simulink model "Electrical_System_2018b_obfs"  (R2019b)
settings: Solver=VariableStepAuto  StartTime=0.0  StopTime=5  RelTol=1e-3  AbsTol=1e-3  EnableMultiTasking=on
InitFcn:
  | Steady_State_Initialisation;
StopFcn:
  | %sscexplore(simlog);
  | %Logging
undefined symbols (not defined in the file): abrlhklxvp, aexgmhuedq, afmfmjnutg, afpphrjpnc, ahuxbyvruc, alarvljztt, amxnyqmnuw, aodrlwvqie, aolhmuplyq, aqpmguuqkg, auesgwirzl, aurophlnng, awamelrhru, ayfhvxflxn, azxkacuhqc, babszerikg, bawhdqanwq, bevoqecvei, bltjvqbchx, bmqsuewujl, bsmyqjfgnf, btvjbsmnve, bywgxqeadw, bziaduxaer, bzmcmdqocb, bzsvyvetat, ccsjnrbsih, cdvenygxwh, cedkrnslhx, cjheorclzs, cjrdshrtqx, ckhavyhcza, ckxewznhlz, cmrcgyiplk, conenicnws, cqkejbgjnn, csfnuwymhe, cunupkhwbh, cwzfvzuxxh, dcadmadufn, dcfponivnv, ddtrqjrhjn, dfhoxvkqas, dfrhtcwpne, dfvomcagjv, djijwylxea, dnmeqksrrm, dnzewbdkaa, dsqcykyxav, dtswwlttmm, ecumpidjtv, edegaywrct, ejjjsmnejc, eknqnehjdz, emvdetzouf, esxbqkbahr, etnkkbreiq, eunoiiiirw, ewewcuedir, fatkfxdhtc ... (+386)
libraries: fl_lib x802, ee_lib x362, fl_ps_legacy_lib x160, nesl_utility x85
(part 4 of 26)

== system Electrical_System_2018b_obfs/Redacted_4814/Redacted_3928/Redacted_4232 ==
  Redacted_1449 : fl_lib/Physical Signals/Sources/PS Constant  constant=eqnibszxct
  Redacted_{2466,4876,8538,9927} (4 alike) : nesl_utility/Solver Configuration  PhysicalDomain=network_engine_domain  SubClassName=solver  LeftPortType=input  RightPortType=generic  Tones=[]  Harmonics=[]  SimulateNoise=off  Profile=off  UseLocalSampling=off  EnableSwitchedLinearOptims=on  FrequencyDomain=off  UseCCode=off  RelTol=0.001  AbsTol=1e-06  MinStep=1e-09  ToWorkspace=off  RevertToSquareIcSolve=off  NumHomotopyIterations=100  PhasorMode=off  PhasorModeNumHarmonics=1  DoDC=off  ResidualTolerance=1e-09  UseLocalSolver=off  LocalSolverChoice=NE_BACKWARD_EULER_ADVANCER  LocalSolverSampleTime=0.001  DoFixedCost=off  MaxNonlinIter=3  MaxModeIter=2  LinearAlgebra=auto  EquationFormulation=NE_TIME_EF  DelaysMemoryBudget=1024  AutomaticFiltering=on  FilteringTimeConstant=0.001  PartitionStorageMethod=AS_NEEDED  PartitionMemoryBudget=1024  PartitionMethod=ROBUST
  Redacted_3160 : fl_lib/Physical Signals/Sources/PS Constant  constant=pqncstflsc
  Redacted_3437 : fl_lib/Mechanical/Mechanical Sources/Ideal Angular Velocity Source
  Redacted_4262 : fl_lib/Physical Signals/Sources/PS Constant  constant=oqqdmjcrcw
  Redacted_4413 : fl_lib/Physical Signals/Sources/PS Constant  constant=hhihvjdfsh
  Redacted_5160 : fl_lib/Mechanical/Mechanical Sources/Ideal Angular Velocity Source
  Redacted_6287 : fl_lib/Mechanical/Rotational Elements/Mechanical Rotational Reference
  Redacted_6471 : fl_lib/Gas/Elements/Controlled Reservoir (G)  area_A=txuumigmxg m^2
      settings: SourceProductName=Simscape  SourceProductBaseCode=SS  InternalSimscapePortConfiguration="{\"Bottom\":[],\"Left\":[{\"id\":\"A\",\"label\":\"A\",\"type\":\"foundation.gas.gas\"}],\"Right\":[{\"id\":\"T_in\",\"label\":\"T\",\"type\":\"input\"},{\"id\":\"p_in\",\"label\":\"P\",\"type\":\"input\"}],\"Top\":[]}"
  Redacted_6500 : fl_lib/Mechanical/Rotational Elements/Mechanical Rotational Reference
  Redacted_6772 : fl_lib/Physical Signals/Sources/PS Constant  constant=ksqpiswnhf
  Redacted_7758 : fl_lib/Gas/Elements/Controlled Reservoir (G)  area_A=bquqgacvwd m^2
      settings: SourceProductName=Simscape  SourceProductBaseCode=SS  InternalSimscapePortConfiguration="{\"Bottom\":[],\"Left\":[{\"id\":\"A\",\"label\":\"A\",\"type\":\"foundation.gas.gas\"}],\"Right\":[{\"id\":\"T_in\",\"label\":\"T\",\"type\":\"input\"},{\"id\":\"p_in\",\"label\":\"P\",\"type\":\"input\"}],\"Top\":[]}"
  Redacted_7870 : fl_lib/Physical Signals/Sources/PS Constant  constant=kaibuegcpr
  Redacted_8727 : PMIOPort  Side=Right
  Redacted_8285 : PMIOPort  Port=2  Side=Right
  Redacted_5217 : PMIOPort  Port=3  Side=Right
  Redacted_9547 : PMIOPort  Port=4  Side=Right
  connections:
  Redacted_3437/LConn1 -- Redacted_4876/RConn1 -- Redacted_5217/RConn1
  Redacted_8727/RConn1 -- Redacted_2466/RConn1 -- Redacted_5160/LConn1
  Redacted_6471/LConn1 -- Redacted_8538/RConn1 -- Redacted_8285/RConn1
  Redacted_9547/RConn1 -- Redacted_9927/RConn1 -- Redacted_7758/LConn1
  Redacted_6500/LConn1 -- Redacted_3437/RConn2
  Redacted_4413/RConn1 -- Redacted_3437/RConn1
  Redacted_5160/RConn1 -- Redacted_3160/RConn1
  Redacted_6287/LConn1 -- Redacted_5160/RConn2
  Redacted_6471/RConn2 -- Redacted_7870/RConn1
  Redacted_6471/RConn1 -- Redacted_4262/RConn1
  Redacted_7758/RConn2 -- Redacted_1449/RConn1
  Redacted_6772/RConn1 -- Redacted_7758/RConn1

== system Electrical_System_2018b_obfs/Redacted_9930/Redacted_3896/Redacted_7665 ==
  Redacted_644 : Outport  InitialOutput=Redacted 0.51183  OutputWhenUnconnectedValue=Redacted 0.067631
  Redacted_2723 : Outport  Port=2  InitialOutput=Redacted 0.06929  OutputWhenUnconnectedValue=Redacted 0.56439
  Redacted_8075 : Outport  Port=3  InitialOutput=Redacted 0.75636  OutputWhenUnconnectedValue=Redacted 0.74779
  Redacted_4126 : Outport  Port=4  InitialOutput=Redacted 0.41895  OutputWhenUnconnectedValue=Redacted 0.34397
  Redacted_7964 : Outport  Port=5  InitialOutput=Redacted 0.88105  OutputWhenUnconnectedValue=Redacted 0.087418
  Redacted_8682 : Outport  Port=6  InitialOutput=Redacted 0.94151  OutputWhenUnconnectedValue=Redacted 0.65364
  Redacted_6320 : Outport  Port=7  InitialOutput=Redacted 0.29985  OutputWhenUnconnectedValue=Redacted 0.09099
  Redacted_340 : Outport  Port=8  InitialOutput=Redacted 0.82117  OutputWhenUnconnectedValue=Redacted 0.22286
  Redacted_2756 : Outport  Port=9  InitialOutput=Redacted 0.3279  OutputWhenUnconnectedValue=Redacted 0.6909
  Redacted_3273 : Outport  Port=10  InitialOutput=Redacted 0.21327  OutputWhenUnconnectedValue=Redacted 0.44752
  Redacted_4657 : Outport  Port=11  InitialOutput=Redacted 0.58417  OutputWhenUnconnectedValue=Redacted 0.30551
  Redacted_3395 : Outport  Port=12  InitialOutput=Redacted 0.23044  OutputWhenUnconnectedValue=Redacted 0.049881
  Redacted_9977 : Outport  Port=13  InitialOutput=Redacted 0.37016  OutputWhenUnconnectedValue=Redacted 0.4867
  Redacted_2599 : Outport  Port=14  InitialOutput=Redacted 0.51394  OutputWhenUnconnectedValue=Redacted 0.10668
  Redacted_1407 : Outport  Port=15  InitialOutput=Redacted 0.046125  OutputWhenUnconnectedValue=Redacted 0.14256
  Redacted_9412 : Outport  Port=16  InitialOutput=Redacted 0.90574  OutputWhenUnconnectedValue=Redacted 0.5736
  Redacted_123 : Outport  Port=17  InitialOutput=Redacted 0.33232  OutputWhenUnconnectedValue=Redacted 0.9768
  Redacted_8209 : Outport  Port=18  InitialOutput=Redacted 0.81768  OutputWhenUnconnectedValue=Redacted 0.20788
  Redacted_531 : Outport  Port=19  InitialOutput=Redacted 0.15823  OutputWhenUnconnectedValue=Redacted 0.1958
  Redacted_6389 : Outport  Port=20  InitialOutput=Redacted 0.98917  OutputWhenUnconnectedValue=Redacted 0.89809
  Redacted_6836 : Outport  Port=21  InitialOutput=Redacted 0.049052  OutputWhenUnconnectedValue=Redacted 0.96153
  Redacted_5007 : Outport  Port=22  InitialOutput=Redacted 0.54549  OutputWhenUnconnectedValue=Redacted 0.87328
  Redacted_6497 : Outport  Port=23  InitialOutput=Redacted 0.97589  OutputWhenUnconnectedValue=Redacted 0.47787
  Redacted_9632 : Outport  Port=24  InitialOutput=Redacted 0.61016  OutputWhenUnconnectedValue=Redacted 0.8766
  Redacted_2902 : Outport  Port=25  InitialOutput=Redacted 0.56898  OutputWhenUnconnectedValue=Redacted 0.30275
  Redacted_2695 : Outport  Port=26  InitialOutput=Redacted 0.96136  OutputWhenUnconnectedValue=Redacted 0.057162
  Redacted_8396 : Outport  Port=27  InitialOutput=Redacted 0.63483  OutputWhenUnconnectedValue=Redacted 0.36709
  Redacted_9164 : Outport  Port=28  InitialOutput=Redacted 0.81001  OutputWhenUnconnectedValue=Redacted 0.29306
  Redacted_9075 : Outport  Port=29  InitialOutput=Redacted 0.54526  OutputWhenUnconnectedValue=Redacted 0.14115
  Redacted_6090 : Outport  Port=30  InitialOutput=Redacted 0.7708  OutputWhenUnconnectedValue=Redacted 0.55418

== system Electrical_System_2018b_obfs/Redacted_9930/Redacted_4814/Redacted_6431 ==
  Redacted_6479 : Outport
  Redacted_3532 : Outport  Port=2
  Redacted_6579 : Outport  Port=3
  Redacted_5091 : Outport  Port=4
  Redacted_5066 : Outport  Port=5
  Redacted_2648 : Outport  Port=6
  Redacted_3799 : Outport  Port=7
  Redacted_988 : Outport  Port=8
  Redacted_4741 : Outport  Port=9
  Redacted_474 : Outport  Port=10
  Redacted_4041 : Outport  Port=11
  Redacted_9998 : Outport  Port=12
  Redacted_2742 : Outport  Port=13
  Redacted_5781 : Outport  Port=14
  Redacted_125 : Outport  Port=15
  Redacted_4308 : Outport  Port=16
  Redacted_8077 : Outport  Port=17
  Redacted_7701 : Outport  Port=18
  Redacted_8967 : Outport  Port=19
  Redacted_8464 : Outport  Port=20
  Redacted_1093 : Outport  Port=21
  Redacted_1950 : Outport  Port=22
  Redacted_1167 : Outport  Port=23
  Redacted_3969 : Outport  Port=24
  Redacted_1905 : Outport  Port=25
  Redacted_1688 : Outport  Port=26
  Redacted_6009 : Outport  Port=27
  Redacted_9612 : Outport  Port=28
  Redacted_8082 : Outport  Port=29
  Redacted_1556 : Outport  Port=30

== system Electrical_System_2018b_obfs/Redacted_1221/Redacted_346/Redacted_2722/Redacted_9748 ==
  note: Transient
  note: Steady-State
  Redacted_8203 : Inport
  Redacted_2737 : Subsystem  VariantControl=Variant1
  Redacted_8358 : PMIOPort  Side=Left
  Redacted_4914 : PMIOPort  Port=2  Side=Left
  Redacted_5870 : PMIOPort  Port=3  Side=Left
  Redacted_79 : PMIOPort  Port=4  Side=Left
  Redacted_7076 : PMIOPort  Port=5  Side=Left
  Redacted_2739 : PMIOPort  Port=6  Side=Left
  Redacted_5893 : PMIOPort  Port=7  Side=Right
  Redacted_5379 : PMIOPort  Port=8  Side=Right
  Redacted_7574 : PMIOPort  Port=9  Side=Right
  Redacted_8270 : PMIOPort  Port=10  Side=Right
  Redacted_8085 : Outport

== system Electrical_System_2018b_obfs/Redacted_1221/Redacted_346/Redacted_3067/Redacted_5519 ==
  note: Steady State
  note: Transient
  Redacted_7936 : Inport
  Redacted_4492 : Subsystem  VariantControl=Choice
  Redacted_7038 : PMIOPort  Side=Right
  Redacted_4138 : PMIOPort  Port=2  Side=Right
  Redacted_4230 : PMIOPort  Port=3  Side=Right
  Redacted_2273 : PMIOPort  Port=4  Side=Left
  Redacted_2496 : PMIOPort  Port=5  Side=Left
  Redacted_4854 : Outport

== system Electrical_System_2018b_obfs/Redacted_1221/Redacted_346/Redacted_5295/Redacted_9981 ==
  note: Steady State
  note: Transient
  Redacted_3927 : Inport
  HP_Generation_Steady_State_Custom_Block : Subsystem  VariantControl=Choice_1
  Redacted_313 : Subsystem  VariantControl=Choice
  Redacted_2793 : PMIOPort  Side=Right
  Redacted_4361 : PMIOPort  Port=2  Side=Right
  Redacted_664 : PMIOPort  Port=3  Side=Right
  Redacted_7849 : PMIOPort  Port=4  Side=Left
  Redacted_6560 : PMIOPort  Port=5  Side=Left
  Redacted_2300 : PMIOPort  Port=6  Side=Left
  Redacted_8917 : PMIOPort  Port=7  Side=Left
  Redacted_8702 : Outport

== system Electrical_System_2018b_obfs/Redacted_1221/Redacted_346/Redacted_6610/Redacted_2835 ==
  note: Steady State
  note: Transient
  Redacted_1740 : Inport
  LP_Generation_Steady_State_Custom_Block : Subsystem  VariantControl=Choice_1
  Redacted_9252 : Subsystem  VariantControl=Choice
  Redacted_9392 : PMIOPort  Side=Right
  Redacted_5211 : PMIOPort  Port=2  Side=Right
  Redacted_1737 : PMIOPort  Port=3  Side=Right
  Redacted_5882 : PMIOPort  Port=4  Side=Left
  Redacted_3815 : PMIOPort  Port=5  Side=Left
  Redacted_3823 : PMIOPort  Port=6  Side=Left
  Redacted_270 : PMIOPort  Port=7  Side=Left
  Redacted_5993 : Outport

== system Electrical_System_2018b_obfs/Redacted_1221/Redacted_7523/Redacted_2432/Redacted_3397 ==
  note: Steady State
  note: Transient
  Redacted_7824 : Inport
  Redacted_440 : Subsystem  VariantControl=Choice
  Redacted_9237 : PMIOPort  Side=Right
  Redacted_7902 : PMIOPort  Port=2  Side=Right
  Redacted_6078 : PMIOPort  Port=3  Side=Right
  Redacted_5254 : PMIOPort  Port=4  Side=Left
  Redacted_3960 : PMIOPort  Port=5  Side=Left
  Redacted_3107 : Outport

== system Electrical_System_2018b_obfs/Redacted_1221/Redacted_7523/Redacted_5456/Redacted_1170 ==
  note: Steady State
  note: Transient
  Redacted_533 : Inport
  HP_Generation_Steady_State_Custom_Block : Subsystem  VariantControl=Choice_1
  Redacted_7838 : Subsystem  VariantControl=Choice
  Redacted_7127 : PMIOPort  Side=Right
  Redacted_9296 : PMIOPort  Port=2  Side=Right
  Redacted_1514 : PMIOPort  Port=3  Side=Right
  Redacted_8915 : PMIOPort  Port=4  Side=Left
  Redacted_4767 : PMIOPort  Port=5  Side=Left
  Redacted_5927 : PMIOPort  Port=6  Side=Left
  Redacted_4590 : PMIOPort  Port=7  Side=Left
  Redacted_7763 : Outport

== system Electrical_System_2018b_obfs/Redacted_1221/Redacted_7523/Redacted_5495/Redacted_794 ==
  note: Steady State
  note: Transient
  Redacted_2518 : Inport
  LP_Generation_Steady_State_Custom_Block : Subsystem  VariantControl=Choice_1
  Redacted_2986 : Subsystem  VariantControl=Choice
  Redacted_4330 : PMIOPort  Side=Right
  Redacted_8728 : PMIOPort  Port=2  Side=Right
  Redacted_6820 : PMIOPort  Port=3  Side=Right
  Redacted_4207 : PMIOPort  Port=4  Side=Left
  Redacted_9340 : PMIOPort  Port=5  Side=Left
  Redacted_923 : PMIOPort  Port=6  Side=Left
  Redacted_1 : PMIOPort  Port=7  Side=Left
  Redacted_6500 : Outport

== system Electrical_System_2018b_obfs/Redacted_1221/Redacted_7523/Redacted_6578/Redacted_4285 ==
  note: Transient
  note: Steady-State
  Redacted_4594 : Inport
  Redacted_3495 : Subsystem  VariantControl=Variant1
  Redacted_9951 : PMIOPort  Side=Left
  Redacted_9283 : PMIOPort  Port=2  Side=Left
  Redacted_674 : PMIOPort  Port=3  Side=Left
  Redacted_4113 : PMIOPort  Port=4  Side=Left
  Redacted_9229 : PMIOPort  Port=5  Side=Left
  Redacted_4224 : PMIOPort  Port=6  Side=Left
  Redacted_5740 : PMIOPort  Port=7  Side=Right
  Redacted_9161 : PMIOPort  Port=8  Side=Right
  Redacted_6949 : PMIOPort  Port=9  Side=Right
  Redacted_5247 : PMIOPort  Port=10  Side=Right
  Redacted_2646 : Outport

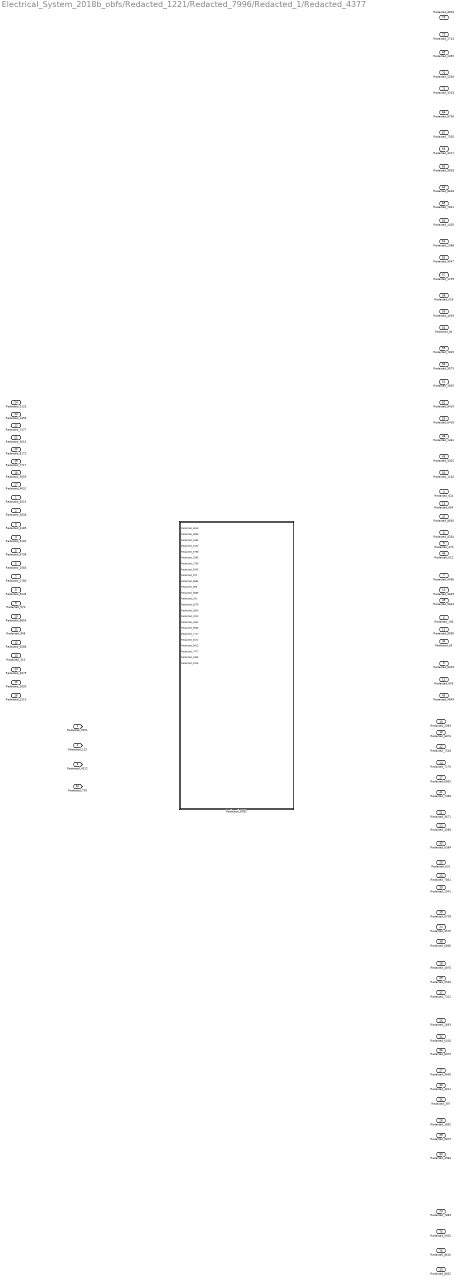
== system Electrical_System_2018b_obfs/Redacted_1221/Redacted_7996/Redacted_1/Redacted_4377 ==
  Redacted_6515 : Inport
  Redacted_5838 : Inport  Port=2
  Redacted_3185 : Inport  Port=3
  Redacted_5102 : Inport  Port=4
  Redacted_6798 : Inport  Port=5
  Redacted_2583 : Inport  Port=6
  Redacted_1780 : Inport  Port=7
  Redacted_5045 : Inport  Port=8
  Redacted_970 : Inport  Port=9
  Redacted_8855 : Inport  Port=10
  Redacted_968 : Inport  Port=11
  Redacted_6586 : Inport  Port=12
  Redacted_310 : Inport  Port=13
  Redacted_3079 : Inport  Port=14
  Redacted_2830 : Inport  Port=15
  Redacted_2310 : Inport  Port=16
  Redacted_4631 : Inport  Port=17
  Redacted_9555 : Inport  Port=18
  Redacted_7717 : Inport  Port=19
  Redacted_8172 : Inport  Port=20
  Redacted_9013 : Inport  Port=21
  Redacted_7477 : Inport  Port=22
  Redacted_1693 : Inport  Port=23
  Redacted_9125 : Inport  Port=24
  Redacted_6082 : Subsystem  VariantControl=Variant4
  Redacted_9251 : PMIOPort  Side=Right
  Redacted_123 : PMIOPort  Port=2  Side=Right
  Redacted_4312 : PMIOPort  Port=3  Side=Right
  Redacted_624 : PMIOPort  Port=4  Side=Right
  Redacted_8329 : PMIOPort  Port=5  Side=Right
  Redacted_196 : PMIOPort  Port=6  Side=Right
  Redacted_4066 : PMIOPort  Port=7  Side=Right
  Redacted_8264 : PMIOPort  Port=8  Side=Right
  Redacted_370 : PMIOPort  Port=9  Side=Right
  Redacted_3639 : PMIOPort  Port=10  Side=Right
  Redacted_8990 : PMIOPort  Port=11  Side=Right
  Redacted_603 : PMIOPort  Port=12  Side=Right
  Redacted_664 : PMIOPort  Port=13  Side=Right
  Redacted_7176 : PMIOPort  Port=14  Side=Right
  Redacted_2083 : PMIOPort  Port=15  Side=Right
  Redacted_6874 : PMIOPort  Port=16  Side=Right
  Redacted_6862 : PMIOPort  Port=17  Side=Right
  Redacted_4876 : PMIOPort  Port=18  Side=Right
  Redacted_6709 : PMIOPort  Port=19  Side=Right
  Redacted_631 : PMIOPort  Port=20  Side=Right
  Redacted_3671 : PMIOPort  Port=21  Side=Right
  Redacted_4589 : PMIOPort  Port=22  Side=Right
  Redacted_7861 : PMIOPort  Port=23  Side=Right
  Redacted_4570 : PMIOPort  Port=24  Side=Right
  Redacted_2535 : PMIOPort  Port=25  Side=Right
  Redacted_2893 : PMIOPort  Port=26  Side=Right
  Redacted_9606 : PMIOPort  Port=27  Side=Right
  Redacted_1862 : PMIOPort  Port=28  Side=Right
  Redacted_9875 : PMIOPort  Port=29  Side=Right
  Redacted_4011 : PMIOPort  Port=30  Side=Right
  Redacted_6416 : PMIOPort  Port=31  Side=Right
  Redacted_705 : PMIOPort  Port=32  Side=Left
  Redacted_8832 : PMIOPort  Port=33  Side=Left
  Redacted_4983 : PMIOPort  Port=34  Side=Left
  Redacted_397 : PMIOPort  Port=35  Side=Left
  Redacted_8070 : PMIOPort  Port=36  Side=Left
  Redacted_7312 : PMIOPort  Port=37  Side=Left
  Redacted_6866 : PMIOPort  Port=38  Side=Left
  Redacted_1941 : PMIOPort  Port=39  Side=Left
  Redacted_6384 : PMIOPort  Port=40  Side=Left
  Redacted_7398 : PMIOPort  Port=41  Side=Left
  Redacted_7548 : PMIOPort  Port=42  Side=Left
  Redacted_4849 : PMIOPort  Port=43  Side=Left
  Redacted_65 : PMIOPort  Port=44  Side=Left
  Redacted_5643 : PMIOPort  Port=45  Side=Left
  Redacted_612 : PMIOPort  Port=46  Side=Left
  Redacted_8660 : PMIOPort  Port=47  Side=Left
  Redacted_1461 : PMIOPort  Port=48  Side=Right
  Redacted_9302 : PMIOPort  Port=49  Side=Right
  Redacted_1140 : PMIOPort  Port=50  Side=Left
  Redacted_3955 : PMIOPort  Port=51  Side=Right
  Redacted_8410 : PMIOPort  Port=52  Side=Right
  Redacted_6418 : PMIOPort  Port=53  Side=Left
  Redacted_84 : PMIOPort  Port=54  Side=Right
  Redacted_7825 : PMIOPort  Port=55  Side=Right
  Redacted_9573 : PMIOPort  Port=56  Side=Left
  Redacted_1199 : PMIOPort  Port=57  Side=Right
  Redacted_518 : PMIOPort  Port=58  Side=Right
  Redacted_4639 : PMIOPort  Port=59  Side=Left
  Redacted_4435 : PMIOPort  Port=60  Side=Right
  Redacted_2388 : PMIOPort  Port=61  Side=Right
  Redacted_9547 : PMIOPort  Port=62  Side=Left
  Redacted_9828 : PMIOPort  Port=63  Side=Right
  Redacted_8618 : PMIOPort  Port=64  Side=Right
  Redacted_7821 : PMIOPort  Port=65  Side=Left
  Redacted_8736 : PMIOPort  Port=66  Side=Right
  Redacted_7335 : PMIOPort  Port=67  Side=Right
  Redacted_3217 : PMIOPort  Port=68  Side=Left
  Redacted_2355 : PMIOPort  Port=69  Side=Right
  Redacted_5260 : PMIOPort  Port=70  Side=Right
  Redacted_9203 : PMIOPort  Port=71  Side=Left
  Redacted_8923 : PMIOPort  Port=72  Side=Right
  Redacted_2743 : PMIOPort  Port=73  Side=Right
  Redacted_7869 : PMIOPort  Port=74  Side=Right
  Redacted_5920 : PMIOPort  Port=75  Side=Right
  Redacted_8610 : PMIOPort  Port=76  Side=Right

== system Electrical_System_2018b_obfs/Redacted_1221/Redacted_7996/Redacted_2/Redacted_38 ==
  Redacted_7517 : Inport
  Redacted_9730 : Inport  Port=2
  Redacted_3026 : Inport  Port=3
  Redacted_8427 : Inport  Port=4
  Redacted_9135 : Inport  Port=5
  Redacted_9726 : Inport  Port=6
  Redacted_8107 : Subsystem  VariantControl=Variant1
  Redacted_2598 : PMIOPort  Side=Left
  Redacted_6678 : PMIOPort  Port=2  Side=Left
  Redacted_3219 : PMIOPort  Port=3  Side=Left
  Redacted_8217 : PMIOPort  Port=4  Side=Left
  Redacted_2962 : PMIOPort  Port=5  Side=Left
  Redacted_1021 : PMIOPort  Port=6  Side=Left
  Redacted_6897 : PMIOPort  Port=7  Side=Right
  Redacted_5408 : PMIOPort  Port=8  Side=Right
  Redacted_5672 : PMIOPort  Port=9  Side=Right
  Redacted_9448 : PMIOPort  Port=10  Side=Left
  Redacted_5088 : PMIOPort  Port=11  Side=Left
  Redacted_6845 : PMIOPort  Port=12  Side=Left
  Redacted_3474 : PMIOPort  Port=13  Side=Left
  Redacted_5409 : PMIOPort  Port=14  Side=Right
  Redacted_5658 : PMIOPort  Port=15  Side=Right
  Redacted_4514 : PMIOPort  Port=16  Side=Right
  Redacted_4323 : PMIOPort  Port=17  Side=Left
  Redacted_5861 : PMIOPort  Port=18  Side=Left
  Redacted_7097 : PMIOPort  Port=19  Side=Left
  Redacted_2682 : PMIOPort  Port=20  Side=Left
  Redacted_548 : PMIOPort  Port=21  Side=Left
  Redacted_1558 : PMIOPort  Port=22  Side=Left

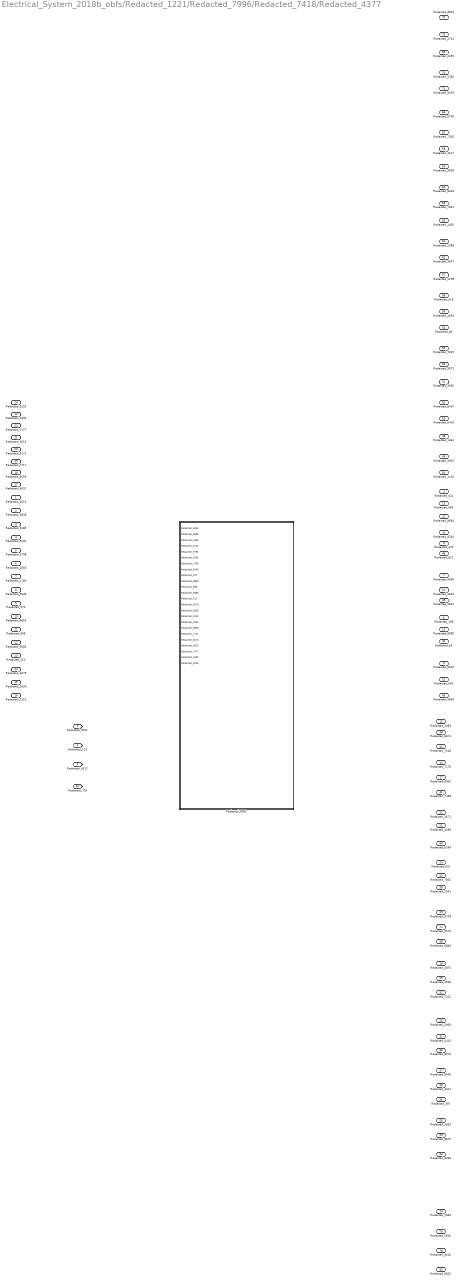
== system Electrical_System_2018b_obfs/Redacted_1221/Redacted_7996/Redacted_7418/Redacted_4377 ==
  Redacted_6515 : Inport
  Redacted_5838 : Inport  Port=2
  Redacted_3185 : Inport  Port=3
  Redacted_5102 : Inport  Port=4
  Redacted_6798 : Inport  Port=5
  Redacted_2583 : Inport  Port=6
  Redacted_1780 : Inport  Port=7
  Redacted_5045 : Inport  Port=8
  Redacted_970 : Inport  Port=9
  Redacted_8855 : Inport  Port=10
  Redacted_968 : Inport  Port=11
  Redacted_6586 : Inport  Port=12
  Redacted_310 : Inport  Port=13
  Redacted_3079 : Inport  Port=14
  Redacted_2830 : Inport  Port=15
  Redacted_2310 : Inport  Port=16
  Redacted_4631 : Inport  Port=17
  Redacted_9555 : Inport  Port=18
  Redacted_7717 : Inport  Port=19
  Redacted_8172 : Inport  Port=20
  Redacted_9013 : Inport  Port=21
  Redacted_7477 : Inport  Port=22
  Redacted_1693 : Inport  Port=23
  Redacted_9125 : Inport  Port=24
  Redacted_6082 : Subsystem  VariantControl=Variant4
  Redacted_9251 : PMIOPort  Side=Right
  Redacted_123 : PMIOPort  Port=2  Side=Right
  Redacted_4312 : PMIOPort  Port=3  Side=Right
  Redacted_624 : PMIOPort  Port=4  Side=Right
  Redacted_8329 : PMIOPort  Port=5  Side=Right
  Redacted_196 : PMIOPort  Port=6  Side=Right
  Redacted_4066 : PMIOPort  Port=7  Side=Right
  Redacted_8264 : PMIOPort  Port=8  Side=Right
  Redacted_370 : PMIOPort  Port=9  Side=Right
  Redacted_3639 : PMIOPort  Port=10  Side=Right
  Redacted_8990 : PMIOPort  Port=11  Side=Right
  Redacted_603 : PMIOPort  Port=12  Side=Right
  Redacted_664 : PMIOPort  Port=13  Side=Right
  Redacted_7176 : PMIOPort  Port=14  Side=Right
  Redacted_2083 : PMIOPort  Port=15  Side=Right
  Redacted_6874 : PMIOPort  Port=16  Side=Right
  Redacted_6862 : PMIOPort  Port=17  Side=Right
  Redacted_4876 : PMIOPort  Port=18  Side=Right
  Redacted_6709 : PMIOPort  Port=19  Side=Right
  Redacted_631 : PMIOPort  Port=20  Side=Right
  Redacted_3671 : PMIOPort  Port=21  Side=Right
  Redacted_4589 : PMIOPort  Port=22  Side=Right
  Redacted_7861 : PMIOPort  Port=23  Side=Right
  Redacted_4570 : PMIOPort  Port=24  Side=Right
  Redacted_2535 : PMIOPort  Port=25  Side=Right
  Redacted_2893 : PMIOPort  Port=26  Side=Right
  Redacted_9606 : PMIOPort  Port=27  Side=Right
  Redacted_1862 : PMIOPort  Port=28  Side=Right
  Redacted_9875 : PMIOPort  Port=29  Side=Right
  Redacted_4011 : PMIOPort  Port=30  Side=Right
  Redacted_6416 : PMIOPort  Port=31  Side=Right
  Redacted_705 : PMIOPort  Port=32  Side=Left
  Redacted_8832 : PMIOPort  Port=33  Side=Left
  Redacted_4983 : PMIOPort  Port=34  Side=Left
  Redacted_397 : PMIOPort  Port=35  Side=Left
  Redacted_8070 : PMIOPort  Port=36  Side=Left
  Redacted_7312 : PMIOPort  Port=37  Side=Left
  Redacted_6866 : PMIOPort  Port=38  Side=Left
  Redacted_1941 : PMIOPort  Port=39  Side=Left
  Redacted_6384 : PMIOPort  Port=40  Side=Left
  Redacted_7398 : PMIOPort  Port=41  Side=Left
  Redacted_7548 : PMIOPort  Port=42  Side=Left
  Redacted_4849 : PMIOPort  Port=43  Side=Left
  Redacted_65 : PMIOPort  Port=44  Side=Left
  Redacted_5643 : PMIOPort  Port=45  Side=Left
  Redacted_612 : PMIOPort  Port=46  Side=Left
  Redacted_8660 : PMIOPort  Port=47  Side=Left
  Redacted_1461 : PMIOPort  Port=48  Side=Right
  Redacted_9302 : PMIOPort  Port=49  Side=Right
  Redacted_1140 : PMIOPort  Port=50  Side=Left
  Redacted_3955 : PMIOPort  Port=51  Side=Right
  Redacted_8410 : PMIOPort  Port=52  Side=Right
  Redacted_6418 : PMIOPort  Port=53  Side=Left
  Redacted_84 : PMIOPort  Port=54  Side=Right
  Redacted_7825 : PMIOPort  Port=55  Side=Right
  Redacted_9573 : PMIOPort  Port=56  Side=Left
  Redacted_1199 : PMIOPort  Port=57  Side=Right
  Redacted_518 : PMIOPort  Port=58  Side=Right
  Redacted_4639 : PMIOPort  Port=59  Side=Left
  Redacted_4435 : PMIOPort  Port=60  Side=Right
  Redacted_2388 : PMIOPort  Port=61  Side=Right
  Redacted_9547 : PMIOPort  Port=62  Side=Left
  Redacted_9828 : PMIOPort  Port=63  Side=Right
  Redacted_8618 : PMIOPort  Port=64  Side=Right
  Redacted_7821 : PMIOPort  Port=65  Side=Left
  Redacted_8736 : PMIOPort  Port=66  Side=Right
  Redacted_7335 : PMIOPort  Port=67  Side=Right
  Redacted_3217 : PMIOPort  Port=68  Side=Left
  Redacted_2355 : PMIOPort  Port=69  Side=Right
  Redacted_5260 : PMIOPort  Port=70  Side=Right
  Redacted_9203 : PMIOPort  Port=71  Side=Left
  Redacted_8923 : PMIOPort  Port=72  Side=Right
  Redacted_2743 : PMIOPort  Port=73  Side=Right
  Redacted_7869 : PMIOPort  Port=74  Side=Right
  Redacted_5920 : PMIOPort  Port=75  Side=Right
  Redacted_8610 : PMIOPort  Port=76  Side=Right

== system Electrical_System_2018b_obfs/Redacted_1221/Redacted_7996/Redacted_9242/Redacted_38 ==
  Redacted_7517 : Inport
  Redacted_9730 : Inport  Port=2
  Redacted_3026 : Inport  Port=3
  Redacted_8427 : Inport  Port=4
  Redacted_9135 : Inport  Port=5
  Redacted_9726 : Inport  Port=6
  Redacted_8107 : Subsystem  VariantControl=Variant1
  Redacted_2598 : PMIOPort  Side=Left
  Redacted_6678 : PMIOPort  Port=2  Side=Left
  Redacted_3219 : PMIOPort  Port=3  Side=Left
  Redacted_8217 : PMIOPort  Port=4  Side=Left
  Redacted_2962 : PMIOPort  Port=5  Side=Left
  Redacted_1021 : PMIOPort  Port=6  Side=Left
  Redacted_6897 : PMIOPort  Port=7  Side=Right
  Redacted_5408 : PMIOPort  Port=8  Side=Right
  Redacted_5672 : PMIOPort  Port=9  Side=Right
  Redacted_9448 : PMIOPort  Port=10  Side=Left
  Redacted_5088 : PMIOPort  Port=11  Side=Left
  Redacted_6845 : PMIOPort  Port=12  Side=Left
  Redacted_3474 : PMIOPort  Port=13  Side=Left
  Redacted_5409 : PMIOPort  Port=14  Side=Right
  Redacted_5658 : PMIOPort  Port=15  Side=Right
  Redacted_4514 : PMIOPort  Port=16  Side=Right
  Redacted_4323 : PMIOPort  Port=17  Side=Left
  Redacted_5861 : PMIOPort  Port=18  Side=Left
  Redacted_7097 : PMIOPort  Port=19  Side=Left
  Redacted_2682 : PMIOPort  Port=20  Side=Left
  Redacted_548 : PMIOPort  Port=21  Side=Left
  Redacted_1558 : PMIOPort  Port=22  Side=Left

== system Electrical_System_2018b_obfs/Redacted_1221/Redacted_346/Redacted_2722/Redacted_9748/Redacted_2737 ==
  Redacted_1110 : fl_lib/Thermal/Thermal Elements/Thermal Reference
  Redacted_{2631,4280,5034,7181} (4 alike) : fl_lib/Electrical/Electrical Sensors/Current Sensor
  Redacted_{2852,7169,7273,9682} (4 alike) : fl_lib/Physical Signals/Sinks/PS Terminator
      settings: SourceProductName=Simscape
  Redacted_4210 : fl_lib/Thermal/Thermal Elements/Thermal Reference
  Redacted_8358 : PMIOPort  Side=Left
  Redacted_4914 : PMIOPort  Port=2  Side=Left
  Redacted_5870 : PMIOPort  Port=3  Side=Left
  Redacted_79 : PMIOPort  Port=4  Side=Left
  Redacted_7076 : PMIOPort  Port=5  Side=Left
  Redacted_2739 : PMIOPort  Port=6  Side=Left
  Redacted_5893 : PMIOPort  Port=7  Side=Right
  Redacted_5379 : PMIOPort  Port=8  Side=Right
  Redacted_7574 : PMIOPort  Port=9  Side=Right
  Redacted_8270 : PMIOPort  Port=10  Side=Right
  connections:
  Redacted_2852/LConn1 -- Redacted_4280/RConn1
  Redacted_7273/LConn1 -- Redacted_2631/RConn1
  Redacted_7181/RConn1 -- Redacted_9682/LConn1
  Redacted_5034/RConn1 -- Redacted_7169/LConn1
  Redacted_5034/RConn2 -- Redacted_5893/RConn1
  Redacted_5034/LConn1 -- Redacted_5870/RConn1
  Redacted_2631/RConn2 -- Redacted_7574/RConn1
  Redacted_2631/LConn1 -- Redacted_7076/RConn1
  Redacted_4280/LConn1 -- Redacted_2739/RConn1
  Redacted_8270/RConn1 -- Redacted_4280/RConn2
  Redacted_7181/RConn2 -- Redacted_5379/RConn1
  Redacted_7181/LConn1 -- Redacted_79/RConn1
  Redacted_8358/RConn1 -- Redacted_1110/LConn1
  Redacted_4914/RConn1 -- Redacted_4210/LConn1

== system Electrical_System_2018b_obfs/Redacted_1221/Redacted_346/Redacted_3067/Redacted_5519/Redacted_4492 ==
  Redacted_5087 : fl_lib/Electrical/Electrical Sources/DC Voltage Source  v0=sdxrqvtcqd V
  Redacted_636 : fl_lib/Electrical/Electrical Sources/DC Voltage Source  v0=mlinvtoslg V
  Redacted_6793 : fl_lib/Thermal/Thermal Elements/Thermal Reference
  Redacted_7322 : fl_lib/Thermal/Thermal Elements/Thermal Reference
  Redacted_7038 : PMIOPort  Side=Right
  Redacted_4138 : PMIOPort  Port=2  Side=Right
  Redacted_4230 : PMIOPort  Port=3  Side=Right
  Redacted_2273 : PMIOPort  Port=4  Side=Left
  Redacted_2496 : PMIOPort  Port=5  Side=Left
  connections:
  Redacted_4138/RConn1 -- Redacted_636/RConn1 -- Redacted_5087/RConn1
  Redacted_2496/RConn1 -- Redacted_7322/LConn1
  Redacted_5087/LConn1 -- Redacted_4230/RConn1
  Redacted_2273/RConn1 -- Redacted_6793/LConn1
  Redacted_7038/RConn1 -- Redacted_636/LConn1

== system Electrical_System_2018b_obfs/Redacted_1221/Redacted_346/Redacted_5295/Redacted_9981/HP_Generation_Steady_State_Custom_Block ==
  Cap (G) : fl_lib/Gas/Elements/Cap (G)  p_specify=off  p_priority=None  p=0.101325 MPa  p_nominal_specify=off  p_nominal_unit=MPa  p_nominal_value=1  T_specify=off  T_priority=None  T=293.15 K  T_nominal_specify=off  T_nominal_unit=K  T_nominal_value=1
      settings: SourceProductName=Simscape  SourceProductBaseCode=SS
  HP Machine and Converter : SimscapeComponentBlock  SourceFile=machine_converter_combination  ComponentPath=machine_converter_combination  ComponentVariants=machine_converter_combination  ComponentVariantNames=machine_converter_combination  ClassName=machine_converter_combination  SchemaVersion=1  pp=5  R=9.9E-3  Ke=0.208 V/rpm  Lq=8.1E-6 H  Ld=8.1E-6 H  num_parallel_modules=4  PWM_F=35000 Hz  Dr=0.198 m  Lact=0.1046 m  DelGap=0.0015 m  NoB=3  Id=0 A
      settings: CopyFcn=simscape.engine.sli.internal.componentblockcallback(gcbh,'COPY')  PreCopyFcn=simscape.engine.sli.internal.componentblockcallback(gcbh,'PRECOPY')  PreDeleteFcn=simscape.engine.sli.internal.componentblockcallback(gcbh,'PREDELETE')  InternalSimscapePortConfiguration="{\"Bottom\":[],\"Left\":[{\"id\":\"Shaft\",\"label\":\"Shaft\",\"type\":\"foundation.mechanical.rotational.rotational\"},{\"id\":\"SAS\",\"label\":\"Air\",\"type\":\"foundation.gas.gas\"}],\"Right\":[{\"id\":\"p\",\"label\":\"+\",\"type\":\"foundation.electrical.electrical\"},{\"id\":\"n\",\"label\":\"-\",\"type\":\"foundation.electrical.electrical\"},{\"id\":\"HC\",\"label\":\"HConverter\",\"type\":\"foundation.thermal.thermal\"},{\"id\":\"HM\",\"label\":\"HMachine\",\"type\":\"foundation.thermal.thermal\"}],\"Top\":[]}"
      mask Type: blah
  HP_Gen+ : fl_lib/Electrical/Electrical Sources/DC Voltage Source  v0=SteadyStateV V
  HP_Gen- : fl_lib/Electrical/Electrical Sources/DC Voltage Source  v0=SteadyStateV V
  Rotational Free End : fl_lib/Mechanical/Rotational Elements/Rotational Free End  w_specify=off  w_priority=None  w=0 rad/s  w_nominal_specify=off  w_nominal_unit=rad/s  w_nominal_value=1
      settings: SourceProductName=Simscape  SourceProductBaseCode=SS
  Redacted_2793 : PMIOPort  Side=Right
  Redacted_4361 : PMIOPort  Port=2  Side=Right
  Redacted_664 : PMIOPort  Port=3  Side=Right
  Redacted_7849 : PMIOPort  Port=4  Side=Left
  Redacted_6560 : PMIOPort  Port=5  Side=Left
  Redacted_2300 : PMIOPort  Port=6  Side=Left
  Redacted_8917 : PMIOPort  Port=7  Side=Left
  connections:
  HP_Gen+/LConn1 -- Redacted_2793/RConn1 -- HP Machine and Converter/RConn1
  HP_Gen-/RConn1 -- Redacted_664/RConn1 -- HP Machine and Converter/RConn2
  HP_Gen+/RConn1 -- Redacted_4361/RConn1 -- HP_Gen-/LConn1
  HP Machine and Converter/LConn2 -- Redacted_6560/RConn1 -- Cap (G)/LConn1
  HP Machine and Converter/LConn1 -- Redacted_7849/RConn1 -- Rotational Free End/LConn1
  Redacted_8917/RConn1 -- HP Machine and Converter/RConn3
  Redacted_2300/RConn1 -- HP Machine and Converter/RConn4

== system Electrical_System_2018b_obfs/Redacted_1221/Redacted_346/Redacted_5295/Redacted_9981/Redacted_313 ==
  Redacted_2067 : fl_lib/Electrical/Electrical Sources/DC Voltage Source  v0=ibzuxmsqbi V
  Redacted_2425 : Subsystem
  Redacted_3600 : fl_lib/Thermal/Thermal Elements/Thermal Reference
  Redacted_4395 : fl_lib/Gas/Elements/Cap (G)  p_specify=off  p_priority=None  p=njgxqsnfqo MPa  p_nominal_specify=off  p_nominal_unit=MPa  p_nominal_value=vcbrpeqxue  T_specify=off  T_priority=None  T=cedkrnslhx K  T_nominal_specify=off  T_nominal_unit=K  T_nominal_value=mgvjnyygja
      settings: SourceProductName=Simscape  SourceProductBaseCode=SS
  Redacted_4714 : fl_lib/Electrical/Electrical Sources/DC Voltage Source  v0=klgonhgwrm V
  Redacted_59 : fl_lib/Mechanical/Rotational Elements/Rotational Free End  w_specify=off  w_priority=None  w=gpbwupqhcq rad/s  w_nominal_specify=off  w_nominal_unit=rad/s  w_nominal_value=dnirxlikvp
      settings: SourceProductName=Simscape  SourceProductBaseCode=SS
  Redacted_6908 : Subsystem
  Redacted_6941 : fl_lib/Thermal/Thermal Elements/Thermal Reference
  Redacted_7365 : Subsystem
  Redacted_2793 : PMIOPort  Side=Right
  Redacted_4361 : PMIOPort  Port=2  Side=Right
  Redacted_664 : PMIOPort  Port=3  Side=Right
  Redacted_2300 : PMIOPort  Port=4  Side=Left
  Redacted_8917 : PMIOPort  Port=5  Side=Left
  Redacted_7849 : PMIOPort  Port=6  Side=Left
  Redacted_6560 : PMIOPort  Port=7  Side=Left
  connections:
  Redacted_6908/RConn1 -- Redacted_7365/RConn1 -- Redacted_2425/RConn1 -- Redacted_2793/RConn1 -- Redacted_2067/LConn1
  Redacted_4714/LConn1 -- Redacted_4361/RConn1 -- Redacted_2067/RConn1
  Redacted_6908/LConn1 -- Redacted_7365/LConn1 -- Redacted_2425/LConn1 -- Redacted_664/RConn1 -- Redacted_4714/RConn1
  Redacted_59/LConn1 -- Redacted_7849/RConn1
  Redacted_2300/RConn1 -- Redacted_3600/LConn1
  Redacted_8917/RConn1 -- Redacted_6941/LConn1
  Redacted_4395/LConn1 -- Redacted_6560/RConn1

== system Electrical_System_2018b_obfs/Redacted_1221/Redacted_346/Redacted_6610/Redacted_2835/LP_Generation_Steady_State_Custom_Block ==
  Cap (G) : fl_lib/Gas/Elements/Cap (G)  p_specify=off  p_priority=None  p=0.101325 MPa  p_nominal_specify=off  p_nominal_unit=MPa  p_nominal_value=1  T_specify=off  T_priority=None  T=293.15 K  T_nominal_specify=off  T_nominal_unit=K  T_nominal_value=1
      settings: SourceProductName=Simscape  SourceProductBaseCode=SS
  HP Machine and Converter : SimscapeComponentBlock  SourceFile=machine_converter_combination  ComponentPath=machine_converter_combination  ComponentVariants=machine_converter_combination  ComponentVariantNames=machine_converter_combination  ClassName=machine_converter_combination  SchemaVersion=1  pp=5  R=9.9E-3  Ke=0.208 V/rpm  Lq=8.1E-6 H  Ld=8.1E-6 H  num_parallel_modules=4  PWM_F=35000 Hz  Dr=0.198 m  Lact=0.1046 m  DelGap=0.0015 m  NoB=3  Id=0 A
      settings: CopyFcn=simscape.engine.sli.internal.componentblockcallback(gcbh,'COPY')  PreCopyFcn=simscape.engine.sli.internal.componentblockcallback(gcbh,'PRECOPY')  PreDeleteFcn=simscape.engine.sli.internal.componentblockcallback(gcbh,'PREDELETE')  InternalSimscapePortConfiguration="{\"Bottom\":[],\"Left\":[{\"id\":\"Shaft\",\"label\":\"Shaft\",\"type\":\"foundation.mechanical.rotational.rotational\"},{\"id\":\"SAS\",\"label\":\"Air\",\"type\":\"foundation.gas.gas\"}],\"Right\":[{\"id\":\"p\",\"label\":\"+\",\"type\":\"foundation.electrical.electrical\"},{\"id\":\"n\",\"label\":\"-\",\"type\":\"foundation.electrical.electrical\"},{\"id\":\"HC\",\"label\":\"HConverter\",\"type\":\"foundation.thermal.thermal\"},{\"id\":\"HM\",\"label\":\"HMachine\",\"type\":\"foundation.thermal.thermal\"}],\"Top\":[]}"
      mask Type: blah
  LP_Gen+ : fl_lib/Electrical/Electrical Sources/DC Voltage Source  v0=SteadyStateV V
  LP_Gen- : fl_lib/Electrical/Electrical Sources/DC Voltage Source  v0=SteadyStateV V
  Rotational Free End : fl_lib/Mechanical/Rotational Elements/Rotational Free End  w_specify=off  w_priority=None  w=0 rad/s  w_nominal_specify=off  w_nominal_unit=rad/s  w_nominal_value=1
      settings: SourceProductName=Simscape  SourceProductBaseCode=SS
  Redacted_9392 : PMIOPort  Side=Right
  Redacted_5211 : PMIOPort  Port=2  Side=Right
  Redacted_1737 : PMIOPort  Port=3  Side=Right
  Nl_Shaft : PMIOPort  Port=4  Side=Left
  Redacted_3815 : PMIOPort  Port=5  Side=Left
  Redacted_3823 : PMIOPort  Port=6  Side=Left
  Redacted_270 : PMIOPort  Port=7  Side=Left
  connections:
  Redacted_5211/RConn1 -- LP_Gen-/LConn1 -- LP_Gen+/RConn1
  Redacted_1737/RConn1 -- HP Machine and Converter/RConn2 -- LP_Gen-/RConn1
  Redacted_9392/RConn1 -- HP Machine and Converter/RConn1 -- LP_Gen+/LConn1
  Redacted_3815/RConn1 -- Cap (G)/LConn1 -- HP Machine and Converter/LConn2
  Nl_Shaft/RConn1 -- Rotational Free End/LConn1 -- HP Machine and Converter/LConn1
  Redacted_270/RConn1 -- HP Machine and Converter/RConn3
  Redacted_3823/RConn1 -- HP Machine and Converter/RConn4

== system Electrical_System_2018b_obfs/Redacted_1221/Redacted_346/Redacted_6610/Redacted_2835/Redacted_9252 ==
  Redacted_1277 : Subsystem
  Redacted_1636 : fl_lib/Thermal/Thermal Elements/Thermal Reference
  Redacted_1750 : fl_lib/Thermal/Thermal Elements/Thermal Reference
  Redacted_2895 : fl_lib/Electrical/Electrical Sources/DC Voltage Source  v0=wxfqsqtroo V
  Redacted_3806 : Subsystem
  Redacted_5568 : Subsystem
  Redacted_5647 : fl_lib/Mechanical/Rotational Elements/Rotational Free End  w_specify=off  w_priority=None  w=zoxqulcmyj rad/s  w_nominal_specify=off  w_nominal_unit=rad/s  w_nominal_value=kseuhykfuc
      settings: SourceProductName=Simscape  SourceProductBaseCode=SS
  Redacted_6009 : fl_lib/Electrical/Electrical Sources/DC Voltage Source  v0=zvkjpexvya V
  Redacted_9116 : fl_lib/Gas/Elements/Cap (G)  p_specify=off  p_priority=None  p=uwjlhbanez MPa  p_nominal_specify=off  p_nominal_unit=MPa  p_nominal_value=pusukhsumo  T_specify=off  T_priority=None  T=svqldgfzpb K  T_nominal_specify=off  T_nominal_unit=K  T_nominal_value=gwwocuxivs
      settings: SourceProductName=Simscape  SourceProductBaseCode=SS
  Redacted_9392 : PMIOPort  Side=Right
  Redacted_5211 : PMIOPort  Port=2  Side=Right
  Redacted_1737 : PMIOPort  Port=3  Side=Right
  Redacted_3823 : PMIOPort  Port=4  Side=Left
  Redacted_270 : PMIOPort  Port=5  Side=Left
  Redacted_5882 : PMIOPort  Port=6  Side=Left
  Redacted_3815 : PMIOPort  Port=7  Side=Left
  connections:
  Redacted_1277/RConn1 -- Redacted_3806/RConn1 -- Redacted_5568/RConn1 -- Redacted_9392/RConn1 -- Redacted_2895/LConn1
  Redacted_6009/LConn1 -- Redacted_5211/RConn1 -- Redacted_2895/RConn1
  Redacted_1277/LConn1 -- Redacted_3806/LConn1 -- Redacted_5568/LConn1 -- Redacted_1737/RConn1 -- Redacted_6009/RConn1
  Redacted_5647/LConn1 -- Redacted_5882/RConn1
  Redacted_9116/LConn1 -- Redacted_3815/RConn1
  Redacted_270/RConn1 -- Redacted_1750/LConn1
  Redacted_3823/RConn1 -- Redacted_1636/LConn1

== system Electrical_System_2018b_obfs/Redacted_1221/Redacted_7523/Redacted_2432/Redacted_3397/Redacted_440 ==
  Redacted_2162 : fl_lib/Electrical/Electrical Sources/DC Voltage Source  v0=pefoovsmtv V
  Redacted_2274 : fl_lib/Thermal/Thermal Elements/Thermal Reference
  Redacted_5384 : fl_lib/Thermal/Thermal Elements/Thermal Reference
  Redacted_5907 : fl_lib/Electrical/Electrical Sources/DC Voltage Source  v0=eigzahxcyb V
  Redacted_9237 : PMIOPort  Side=Right
  Redacted_7902 : PMIOPort  Port=2  Side=Right
  Redacted_6078 : PMIOPort  Port=3  Side=Right
  Redacted_5254 : PMIOPort  Port=4  Side=Left
  Redacted_3960 : PMIOPort  Port=5  Side=Left
  connections:
  Redacted_7902/RConn1 -- Redacted_2162/RConn1 -- Redacted_5907/RConn1
  Redacted_3960/RConn1 -- Redacted_5384/LConn1
  Redacted_5907/LConn1 -- Redacted_6078/RConn1
  Redacted_5254/RConn1 -- Redacted_2274/LConn1
  Redacted_9237/RConn1 -- Redacted_2162/LConn1

== system Electrical_System_2018b_obfs/Redacted_1221/Redacted_7523/Redacted_5456/Redacted_1170/HP_Generation_Steady_State_Custom_Block ==
  Cap (G) : fl_lib/Gas/Elements/Cap (G)  p_specify=off  p_priority=None  p=0.101325 MPa  p_nominal_specify=off  p_nominal_unit=MPa  p_nominal_value=1  T_specify=off  T_priority=None  T=293.15 K  T_nominal_specify=off  T_nominal_unit=K  T_nominal_value=1
      settings: SourceProductName=Simscape  SourceProductBaseCode=SS
  HP Machine and Converter : SimscapeComponentBlock  SourceFile=machine_converter_combination  ComponentPath=machine_converter_combination  ComponentVariants=machine_converter_combination  ComponentVariantNames=machine_converter_combination  ClassName=machine_converter_combination  SchemaVersion=1  pp=5  R=9.9E-3  Ke=0.208 V/rpm  Lq=8.1E-6 H  Ld=8.1E-6 H  num_parallel_modules=4  PWM_F=35000 Hz  Dr=0.198 m  Lact=0.1046 m  DelGap=0.0015 m  NoB=3  Id=0 A
      settings: CopyFcn=simscape.engine.sli.internal.componentblockcallback(gcbh,'COPY')  PreCopyFcn=simscape.engine.sli.internal.componentblockcallback(gcbh,'PRECOPY')  PreDeleteFcn=simscape.engine.sli.internal.componentblockcallback(gcbh,'PREDELETE')  InternalSimscapePortConfiguration="{\"Bottom\":[],\"Left\":[{\"id\":\"Shaft\",\"label\":\"Shaft\",\"type\":\"foundation.mechanical.rotational.rotational\"},{\"id\":\"SAS\",\"label\":\"Air\",\"type\":\"foundation.gas.gas\"}],\"Right\":[{\"id\":\"p\",\"label\":\"+\",\"type\":\"foundation.electrical.electrical\"},{\"id\":\"n\",\"label\":\"-\",\"type\":\"foundation.electrical.electrical\"},{\"id\":\"HC\",\"label\":\"HConverter\",\"type\":\"foundation.thermal.thermal\"},{\"id\":\"HM\",\"label\":\"HMachine\",\"type\":\"foundation.thermal.thermal\"}],\"Top\":[]}"
      mask Type: blah
  HP_Gen+ : fl_lib/Electrical/Electrical Sources/DC Voltage Source  v0=SteadyStateV V
  HP_Gen- : fl_lib/Electrical/Electrical Sources/DC Voltage Source  v0=SteadyStateV V
  Rotational Free End : fl_lib/Mechanical/Rotational Elements/Rotational Free End  w_specify=off  w_priority=None  w=0 rad/s  w_nominal_specify=off  w_nominal_unit=rad/s  w_nominal_value=1
      settings: SourceProductName=Simscape  SourceProductBaseCode=SS
  Redacted_7127 : PMIOPort  Side=Right
  Redacted_9296 : PMIOPort  Port=2  Side=Right
  Redacted_1514 : PMIOPort  Port=3  Side=Right
  Redacted_8915 : PMIOPort  Port=4  Side=Left
  Redacted_4767 : PMIOPort  Port=5  Side=Left
  Redacted_5927 : PMIOPort  Port=6  Side=Left
  Redacted_4590 : PMIOPort  Port=7  Side=Left
  connections:
  HP_Gen+/LConn1 -- Redacted_7127/RConn1 -- HP Machine and Converter/RConn1
  HP_Gen-/RConn1 -- Redacted_1514/RConn1 -- HP Machine and Converter/RConn2
  HP_Gen+/RConn1 -- Redacted_9296/RConn1 -- HP_Gen-/LConn1
  HP Machine and Converter/LConn2 -- Redacted_4767/RConn1 -- Cap (G)/LConn1
  HP Machine and Converter/LConn1 -- Redacted_8915/RConn1 -- Rotational Free End/LConn1
  Redacted_4590/RConn1 -- HP Machine and Converter/RConn3
  Redacted_5927/RConn1 -- HP Machine and Converter/RConn4

== system Electrical_System_2018b_obfs/Redacted_1221/Redacted_7523/Redacted_5456/Redacted_1170/Redacted_7838 ==
  Redacted_1138 : fl_lib/Thermal/Thermal Elements/Thermal Reference
  Redacted_1766 : fl_lib/Gas/Elements/Cap (G)  p_specify=off  p_priority=None  p=dwnzyjzcno MPa  p_nominal_specify=off  p_nominal_unit=MPa  p_nominal_value=lfhawvtcmn  T_specify=off  T_priority=None  T=xlobrkpcch K  T_nominal_specify=off  T_nominal_unit=K  T_nominal_value=cogkmcujvd
      settings: SourceProductName=Simscape  SourceProductBaseCode=SS
  Redacted_2834 : fl_lib/Electrical/Electrical Sources/DC Voltage Source  v0=ytmhctjoad V
  Redacted_5144 : Subsystem
  Redacted_6401 : fl_lib/Mechanical/Rotational Elements/Rotational Free End  w_specify=off  w_priority=None  w=meptlpmiiw rad/s  w_nominal_specify=off  w_nominal_unit=rad/s  w_nominal_value=qiuwyzkkat
      settings: SourceProductName=Simscape  SourceProductBaseCode=SS
  Redacted_7521 : fl_lib/Electrical/Electrical Sources/DC Voltage Source  v0=gixshljbeu V
  Redacted_8977 : Subsystem
  Redacted_9032 : Subsystem
  Redacted_9366 : fl_lib/Thermal/Thermal Elements/Thermal Reference
  Redacted_7127 : PMIOPort  Side=Right
  Redacted_9296 : PMIOPort  Port=2  Side=Right
  Redacted_1514 : PMIOPort  Port=3  Side=Right
  Redacted_5927 : PMIOPort  Port=4  Side=Left
  Redacted_4590 : PMIOPort  Port=5  Side=Left
  Redacted_8915 : PMIOPort  Port=6  Side=Left
  Redacted_4767 : PMIOPort  Port=7  Side=Left
  connections:
  Redacted_9032/RConn1 -- Redacted_5144/RConn1 -- Redacted_8977/RConn1 -- Redacted_7127/RConn1 -- Redacted_7521/LConn1
  Redacted_2834/LConn1 -- Redacted_9296/RConn1 -- Redacted_7521/RConn1
  Redacted_9032/LConn1 -- Redacted_5144/LConn1 -- Redacted_8977/LConn1 -- Redacted_1514/RConn1 -- Redacted_2834/RConn1
  Redacted_6401/LConn1 -- Redacted_8915/RConn1
  Redacted_5927/RConn1 -- Redacted_9366/LConn1
  Redacted_4590/RConn1 -- Redacted_1138/LConn1
  Redacted_1766/LConn1 -- Redacted_4767/RConn1

== system Electrical_System_2018b_obfs/Redacted_1221/Redacted_7523/Redacted_5495/Redacted_794/LP_Generation_Steady_State_Custom_Block ==
  Cap (G) : fl_lib/Gas/Elements/Cap (G)  p_specify=off  p_priority=None  p=0.101325 MPa  p_nominal_specify=off  p_nominal_unit=MPa  p_nominal_value=1  T_specify=off  T_priority=None  T=293.15 K  T_nominal_specify=off  T_nominal_unit=K  T_nominal_value=1
      settings: SourceProductName=Simscape  SourceProductBaseCode=SS
  HP Machine and Converter : SimscapeComponentBlock  SourceFile=machine_converter_combination  ComponentPath=machine_converter_combination  ComponentVariants=machine_converter_combination  ComponentVariantNames=machine_converter_combination  ClassName=machine_converter_combination  SchemaVersion=1  pp=5  R=9.9E-3  Ke=0.208 V/rpm  Lq=8.1E-6 H  Ld=8.1E-6 H  num_parallel_modules=4  PWM_F=35000 Hz  Dr=0.198 m  Lact=0.1046 m  DelGap=0.0015 m  NoB=3  Id=0 A
      settings: CopyFcn=simscape.engine.sli.internal.componentblockcallback(gcbh,'COPY')  PreCopyFcn=simscape.engine.sli.internal.componentblockcallback(gcbh,'PRECOPY')  PreDeleteFcn=simscape.engine.sli.internal.componentblockcallback(gcbh,'PREDELETE')  InternalSimscapePortConfiguration="{\"Bottom\":[],\"Left\":[{\"id\":\"Shaft\",\"label\":\"Shaft\",\"type\":\"foundation.mechanical.rotational.rotational\"},{\"id\":\"SAS\",\"label\":\"Air\",\"type\":\"foundation.gas.gas\"}],\"Right\":[{\"id\":\"p\",\"label\":\"+\",\"type\":\"foundation.electrical.electrical\"},{\"id\":\"n\",\"label\":\"-\",\"type\":\"foundation.electrical.electrical\"},{\"id\":\"HC\",\"label\":\"HConverter\",\"type\":\"foundation.thermal.thermal\"},{\"id\":\"HM\",\"label\":\"HMachine\",\"type\":\"foundation.thermal.thermal\"}],\"Top\":[]}"
      mask Type: blah
  LP_Gen+ : fl_lib/Electrical/Electrical Sources/DC Voltage Source  v0=SteadyStateV V
  LP_Gen- : fl_lib/Electrical/Electrical Sources/DC Voltage Source  v0=SteadyStateV V
  Rotational Free End : fl_lib/Mechanical/Rotational Elements/Rotational Free End  w_specify=off  w_priority=None  w=0 rad/s  w_nominal_specify=off  w_nominal_unit=rad/s  w_nominal_value=1
      settings: SourceProductName=Simscape  SourceProductBaseCode=SS
  Redacted_4330 : PMIOPort  Side=Right
  Redacted_8728 : PMIOPort  Port=2  Side=Right
  Redacted_6820 : PMIOPort  Port=3  Side=Right
  Nl_Shaft : PMIOPort  Port=4  Side=Left
  Redacted_9340 : PMIOPort  Port=5  Side=Left
  Redacted_923 : PMIOPort  Port=6  Side=Left
  Redacted_1 : PMIOPort  Port=7  Side=Left
  connections:
  Redacted_8728/RConn1 -- LP_Gen-/LConn1 -- LP_Gen+/RConn1
  Redacted_6820/RConn1 -- HP Machine and Converter/RConn2 -- LP_Gen-/RConn1
  Redacted_4330/RConn1 -- HP Machine and Converter/RConn1 -- LP_Gen+/LConn1
  Redacted_9340/RConn1 -- Cap (G)/LConn1 -- HP Machine and Converter/LConn2
  Nl_Shaft/RConn1 -- Rotational Free End/LConn1 -- HP Machine and Converter/LConn1
  Redacted_1/RConn1 -- HP Machine and Converter/RConn3
  Redacted_923/RConn1 -- HP Machine and Converter/RConn4

== system Electrical_System_2018b_obfs/Redacted_1221/Redacted_7523/Redacted_5495/Redacted_794/Redacted_2986 ==
  Redacted_113 : fl_lib/Mechanical/Rotational Elements/Rotational Free End  w_specify=off  w_priority=None  w=wusjvwiwzc rad/s  w_nominal_specify=off  w_nominal_unit=rad/s  w_nominal_value=ngzvzialud
      settings: SourceProductName=Simscape  SourceProductBaseCode=SS
  Redacted_177 : Subsystem
  Redacted_3587 : Subsystem
  Redacted_5042 : fl_lib/Electrical/Electrical Sources/DC Voltage Source  v0=sqmblvbsbr V
  Redacted_5184 : fl_lib/Thermal/Thermal Elements/Thermal Reference
  Redacted_7314 : fl_lib/Gas/Elements/Cap (G)  p_specify=off  p_priority=None  p=etojkhznis MPa  p_nominal_specify=off  p_nominal_unit=MPa  p_nominal_value=waialzhygn  T_specify=off  T_priority=None  T=fyikmyqztg K  T_nominal_specify=off  T_nominal_unit=K  T_nominal_value=lrxnavlmzj
      settings: SourceProductName=Simscape  SourceProductBaseCode=SS
  Redacted_7383 : fl_lib/Thermal/Thermal Elements/Thermal Reference
  Redacted_9599 : Subsystem
  Redacted_980 : fl_lib/Electrical/Electrical Sources/DC Voltage Source  v0=wdxoquzfnn V
  Redacted_4330 : PMIOPort  Side=Right
  Redacted_8728 : PMIOPort  Port=2  Side=Right
  Redacted_6820 : PMIOPort  Port=3  Side=Right
  Redacted_923 : PMIOPort  Port=4  Side=Left
  Redacted_1 : PMIOPort  Port=5  Side=Left
  Redacted_4207 : PMIOPort  Port=6  Side=Left
  Redacted_9340 : PMIOPort  Port=7  Side=Left
  connections:
  Redacted_3587/RConn1 -- Redacted_177/RConn1 -- Redacted_9599/RConn1 -- Redacted_4330/RConn1 -- Redacted_980/LConn1
  Redacted_5042/LConn1 -- Redacted_8728/RConn1 -- Redacted_980/RConn1
  Redacted_3587/LConn1 -- Redacted_177/LConn1 -- Redacted_9599/LConn1 -- Redacted_6820/RConn1 -- Redacted_5042/RConn1
  Redacted_113/LConn1 -- Redacted_4207/RConn1
  Redacted_7314/LConn1 -- Redacted_9340/RConn1
  Redacted_1/RConn1 -- Redacted_5184/LConn1
  Redacted_923/RConn1 -- Redacted_7383/LConn1
